simulink model "black_box_ex7"  (Simulink 7.4)
settings: Solver=VariableStepDiscrete  SolverMode=SingleTasking  StartTime=0.0  StopTime=im_size*im_size+40  RelTol=1e-3
PreLoadFcn:
  | black_box_ex7_PreLoadFcn
StopFcn:
  | black_box_ex7_StopFcn
libraries: xbsIndex_r4 x17, xbsCopyrightNotice_r4 x1
settings Model: Creator=vanessay  LastModifiedBy=douangp
settings OptimizationCC: InlineParams=on  InitFltsAndDblsToZero=on

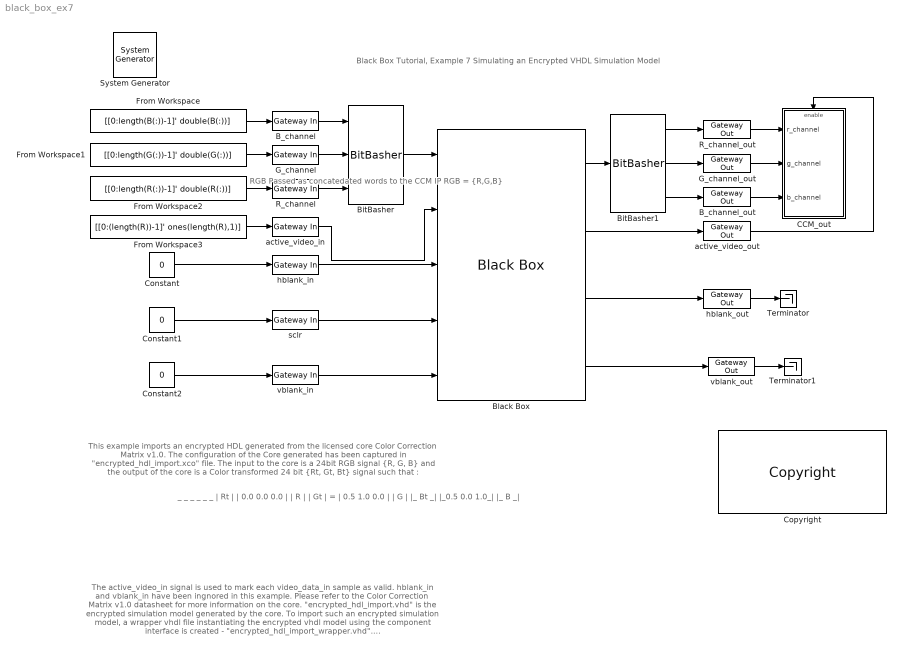
== system black_box_ex7 ==
  note: RGB Passed
      | as concatedated
      | words to the
      | CCM IP
      | RGB = {R,G,B}
  note: Black Box Tutorial, Example 7
      | Simulating an Encrypted VHDL Simulation Model
  note: This example imports an encrypted HDL generated from the licensed core Color Correction Matrix v1.0.
      | The configuration of the Core generated has been captured in "encrypted_hdl_import.xco" file. The input
      | to the core is a 24bit RGB signal {R, G, B} and the output of the core is a Color transformed 24 bit
      | {Rt, Gt, Bt} signal such that :
  note: _    _     _           _   _   _
      | |  Rt  |   | 0.0 0.0 0.0 | |  R  |
      | |  Gt  | = | 0.5 1.0 0.0 | |  G  |
      | |_ Bt _|   |_0.5 0.0 1.0_| |_ B _|
  note: The active_video_in signal is used to mark each video_data_in sample as valid. hblank_in and vblank_in
      | have been ingnored in this example. Please refer to the Color Correction Matrix v1.0 datasheet for more
      | information on the core.
      |
      | "encrypted_hdl_import.vhd" is the encrypted simulation model generated by the core. To import such an
      | encrypted simulation model, a wrapper vhdl file instantiating the encrypted vhdl model using the component
      | interface is created - "encrypted_hdl_import_wrapper.vhd". "encrypted_hdl_import_wrapper.vhd" is imported
      | using the standard Black Box import Wizard. The resulting "encrypted_hdl_import_wrapper_config.m" is
      | modified by adding the following line(line No. 103) :
      |                 this_block.addFile('encrypted_hdl_import.vhd','encrypted_hdl_import.vhd');
      | The above line instructs the SysGen netlister to netlist the encrypted file as a Separate file and not include it
      | in the consolidated HDL netlist file to allow participation of the encrypted HDL file during netlisting and simulation.
  " System Generator" : xbsIndex_r4/ System Generator  Tag=genX  SystemSampleTime=-1  xilinxfamily=spartan3adsp  part=xc3sd3400a  speed=-4  package=fg676  synthesis_tool=XST  clock_wrapper=Clock Enables  directory=./hdl  testbench=off  simulink_period=1  sysclk_period=6.6  dcm_input_clock_period=100  incr_netlist=off  trim_vbits=Everywhere in SubSystem  dbl_ovrd=According to Block Masks  core_generation=According to Block Masks  run_coregen=off  deprecated_control=off  eval_field=0  block_type=sysgen
      settings: block_version=8.2
  B_channel : xbsIndex_r4/Gateway In  arith_type=Unsigned  n_bits=8  bin_pt=0  quantization=Truncate  overflow=Wrap  period=1  dbl_ovrd=off  timing_constraint=None  locs_specified=off  LOCs={}  hdl_port=on  block_type=gatewayin
      settings: infoedit="Gateway in block.  Converts inputs of type Simulink integer, double and fixed point to  Xilinx fixed point type.<br><br>Hardware notes:  In hardware these blocks become top level input ports."  xl_area=[0, 0, 0, 0, 0, 0, 0]  block_version=VER_STRING_GOES_HERE
  B_channel_out : xbsIndex_r4/Gateway Out  hdl_port=on  timing_constraint=None  locs_specified=off  LOCs={}  block_type=gatewayout
      settings: infoedit="Gateway out block.  Converts Xilinx fixed point inputs into ouputs of type Simulink integer, double, or fixed point.<P><P>Hardware notes:  In hardware these blocks become top level output ports or are discarded, depending on how they are configured."  xl_area=[0, 0, 0, 0, 0, 0, 0]  block_version=VER_STRING_GOES_HERE
  BitBasher : xbsIndex_r4/BitBasher  bitexpr=|  display_expr=off  sr_1=1  arith_type1=Unsigned  bin_pt1=0  sr_2=2  arith_type2=Unsigned  bin_pt2=0  sr_3=3  arith_type3=Unsigned  bin_pt3=0  sr_4=4  arith_type4=Unsigned  bin_pt4=0  dbl_ovrd=off  block_type=bitbasher
      | <!DOCTYPE HTML PUBLIC "-//W3C//DTD HTML 4.0//EN" "http://www.w3.org/TR/REC-html40/strict.dtd">
      | <html><head><meta name="qrichtext" content="1" /><style type="text/css">
      | p, li { white-space: pre-wrap; }
      | </style></head><body style=" font-family:'MS Shell Dlg 2'; font-size:8.25pt; font-weight:400; font-style:normal;">
      | <p style=" margin-top:12px; margin-bottom:12px; margin-left:0px; margin-right:0px; -qt-block-indent:0; text-indent:0px; font-family:'MS Shell Dlg'; font-size:8pt;">RGB={R,G,B}</p></body></html>
      settings: block_version=11.3
  BitBasher1 : xbsIndex_r4/BitBasher  bitexpr=|  display_expr=off  sr_1=1  arith_type1=Unsigned  bin_pt1=0  sr_2=2  arith_type2=Unsigned  bin_pt2=0  sr_3=3  arith_type3=Unsigned  bin_pt3=0  sr_4=4  arith_type4=Unsigned  bin_pt4=0  dbl_ovrd=off  block_type=bitbasher
      | <!DOCTYPE HTML PUBLIC "-//W3C//DTD HTML 4.0//EN" "http://www.w3.org/TR/REC-html40/strict.dtd">
      | <html><head><meta name="qrichtext" content="1" /><style type="text/css">
      | p, li { white-space: pre-wrap; }
      | </style></head><body style=" font-family:'MS Shell Dlg 2'; font-size:8.25pt; font-weight:400; font-style:normal;">
      | <p style=" margin-top:12px; margin-bottom:12px; margin-left:0px; margin-right:0px; -qt-block-indent:0; text-indent:0px; font-family:'MS Shell Dlg'; font-size:8pt;">R={RGB[23:16]}<br />G={RGB[15:8]}<br />B={RGB[7:0]}</p></body></html>
      settings: block_version=11.3
  Black Box : xbsIndex_r4/Black Box  init_code=encrypted_hdl_import_wrapper_config  sim_method=ISE Simulator  verbose=off  block_type=blackbox2
      settings: block_version=11.3
  CCM_out : Subsystem  TreatAsAtomicUnit=on
  Constant : Constant  Value=0  OutDataType=sfix(16)  OutScaling=2^0
  Constant1 : Constant  Value=0  OutDataType=sfix(16)  OutScaling=2^0
  Constant2 : Constant  Value=0  OutDataType=sfix(16)  OutScaling=2^0
  Copyright : xbsCopyrightNotice_r4/Copyright  copyrighttext="Copyright (c) 2010  by  Xilinx, Inc. All rights reserved.<br><br>This file contains proprietary, confidential information of Xilinx, Inc., is distributed under licensefrom Xilinx, Inc., and may be used, copied and/or disclosed only pursuant to the terms of a valid licenseagreement with Xilinx, Inc. Xilinx hereby grants you a license to use this file solely for design,simulation, implementation and creation of design files limited to Xilinx devices or technologies. Use with non-Xilinx devices or technologies is expressly prohibited and immediately terminates your license unless covered by a separate agreement.<br><br>Xilinx is providing this design, code, or information \"as-is\" solely for use in developing programs and solutions for Xilinx devices, with no obligation on the part of Xilinx to provide support. By providingthis design, code, or information as one possible implementation of this feature, application or standard,Xilinx is making no representation that this implementation is free from any claims of infringement. Youare responsible for obtaining any rights you may require for your implementation. Xilinx expressly disclaimsany warranty whatsoever with respect to the adequacy of the implementation, including but not limited to anywarranties or representations that this implementation is free from claims of infringement, implied warrantiesof merchantability or fitness for a particular purpose.<br><br>Xilinx products are not intended for use in life support appliances, devices, or systems. Use in such applications is expressly prohibited.<br><br>Any modifications that are made to the Source Code are done at the user's sole risk and will be unsupported.<br><br>This copyright and support notice must be retained as part of this text at all times. (c) Copyright 1995-2010 Xilinx, Inc. All rights reserved."  block_type=copyright
      settings: block_version=10.1.3
      settings: infoedit=|
      | Copyright(C) 2008 by  Xilinx, Inc. All rights reserved.<br>
      | <br>
      | This file contains proprietary, confidential information of Xilinx, Inc., is distributed under license
      | from Xilinx, Inc., and may be used, copied and/or disclosed only pursuant to the terms of a valid license
      | agreement with Xilinx, Inc. Xilinx hereby grants you a license to use this file solely for design,
      | simulation, implementation and creation of design files limited to Xilinx devices or technologies. Use
      | with non-Xilinx devices or technologies is expressly prohibited and immediately terminates your license
      | unless covered by a separate agreement.<br>
      | <br>
      | Xilinx is providing this design, code, or information "as-is" solely for use in developing programs and
      | solutions for Xilinx devices, with no obligation on the part of Xilinx to provide support. By providing
      | this design, code, or information as one possible implementation of this feature, application or standard,
      | Xilinx is making no representation that this implementation is free from any claims of infringement. You
      | are responsible for obtaining any rights you may require for your implementation. Xilinx expressly disclaims
      | any warranty whatsoever with respect to the adequacy of the implementation, including but not limited to any
      | warranties or representations that this implementation is free from claims of infringement, implied warranties
      | of merchantability or fitness for a particular purpose.<br>
      | <br>
      | Xilinx products are not intended for use in life support appliances, devices, or systems. Use in such
      | applications is expressly prohibited.<br>
      | <br>
      | Any modifications that are made to the Source Code are done at the user's sole risk and will be unsupported.<br>
      | <br>
      | This copyright and support notice must be retained as part of this text at all times.
      | (c) Copyright 1995-2008 Xilinx, Inc. All rights reserved.
  From Workspace : FromWorkspace  VariableName=[[0:length(B(:))-1]' double(B(:))]  SampleTime=1
  From Workspace1 : FromWorkspace  VariableName=[[0:length(G(:))-1]' double(G(:))]  SampleTime=1
  From Workspace2 : FromWorkspace  VariableName=[[0:length(R(:))-1]' double(R(:))]  SampleTime=1
  From Workspace3 : FromWorkspace  VariableName=[[0:(length(R))-1]' ones(length(R),1)]  SampleTime=1  OutputAfterFinalValue=Setting to zero
  G_channel : xbsIndex_r4/Gateway In  arith_type=Unsigned  n_bits=8  bin_pt=0  quantization=Truncate  overflow=Wrap  period=1  dbl_ovrd=off  timing_constraint=None  locs_specified=off  LOCs={}  hdl_port=on  block_type=gatewayin
      settings: infoedit="Gateway in block.  Converts inputs of type Simulink integer, double and fixed point to  Xilinx fixed point type.<br><br>Hardware notes:  In hardware these blocks become top level input ports."  xl_area=[0, 0, 0, 0, 0, 0, 0]  block_version=VER_STRING_GOES_HERE
  G_channel_out : xbsIndex_r4/Gateway Out  hdl_port=on  timing_constraint=None  locs_specified=off  LOCs={}  block_type=gatewayout
      settings: infoedit="Gateway out block.  Converts Xilinx fixed point inputs into ouputs of type Simulink integer, double, or fixed point.<P><P>Hardware notes:  In hardware these blocks become top level output ports or are discarded, depending on how they are configured."  xl_area=[0, 0, 0, 0, 0, 0, 0]  block_version=VER_STRING_GOES_HERE
  R_channel : xbsIndex_r4/Gateway In  arith_type=Unsigned  n_bits=8  bin_pt=0  quantization=Truncate  overflow=Wrap  period=1  dbl_ovrd=off  timing_constraint=None  locs_specified=off  LOCs={}  hdl_port=on  block_type=gatewayin
      settings: infoedit="Gateway in block.  Converts inputs of type Simulink integer, double and fixed point to  Xilinx fixed point type.<br><br>Hardware notes:  In hardware these blocks become top level input ports."  xl_area=[0, 0, 0, 0, 0, 0, 0]  block_version=VER_STRING_GOES_HERE
  R_channel_out : xbsIndex_r4/Gateway Out  hdl_port=on  timing_constraint=None  locs_specified=off  LOCs={}  block_type=gatewayout
      settings: infoedit="Gateway out block.  Converts Xilinx fixed point inputs into ouputs of type Simulink integer, double, or fixed point.<P><P>Hardware notes:  In hardware these blocks become top level output ports or are discarded, depending on how they are configured."  xl_area=[0, 0, 0, 0, 0, 0, 0]  block_version=VER_STRING_GOES_HERE
  Terminator : Terminator
  Terminator1 : Terminator
  active_video_in : xbsIndex_r4/Gateway In  arith_type=Unsigned  n_bits=1  bin_pt=0  quantization=Truncate  overflow=Wrap  period=1  dbl_ovrd=off  timing_constraint=None  locs_specified=off  LOCs={}  hdl_port=on  block_type=gatewayin
      settings: infoedit="Gateway in block.  Converts inputs of type Simulink integer, double and fixed point to  Xilinx fixed point type.<br><br>Hardware notes:  In hardware these blocks become top level input ports."  xl_area=[0, 0, 0, 0, 0, 0, 0]  block_version=VER_STRING_GOES_HERE
  active_video_out : xbsIndex_r4/Gateway Out  hdl_port=on  timing_constraint=None  locs_specified=off  LOCs={}  block_type=gatewayout
      settings: infoedit="Gateway out block.  Converts Xilinx fixed point inputs into ouputs of type Simulink integer, double, or fixed point.<P><P>Hardware notes:  In hardware these blocks become top level output ports or are discarded, depending on how they are configured."  xl_area=[0, 0, 0, 0, 0, 0, 0]  block_version=VER_STRING_GOES_HERE
  hblank_in : xbsIndex_r4/Gateway In  arith_type=Unsigned  n_bits=1  bin_pt=0  quantization=Truncate  overflow=Wrap  period=1  dbl_ovrd=off  timing_constraint=None  locs_specified=off  LOCs={}  hdl_port=on  block_type=gatewayin
      settings: infoedit="Gateway in block.  Converts inputs of type Simulink integer, double and fixed point to  Xilinx fixed point type.<br><br>Hardware notes:  In hardware these blocks become top level input ports."  xl_area=[0, 0, 0, 0, 0, 0, 0]  block_version=VER_STRING_GOES_HERE
  hblank_out : xbsIndex_r4/Gateway Out  hdl_port=on  timing_constraint=None  locs_specified=off  LOCs={}  block_type=gatewayout
      settings: infoedit="Gateway out block.  Converts Xilinx fixed point inputs into ouputs of type Simulink integer, double, or fixed point.<P><P>Hardware notes:  In hardware these blocks become top level output ports or are discarded, depending on how they are configured."  xl_area=[0, 0, 0, 0, 0, 0, 0]  block_version=VER_STRING_GOES_HERE
  sclr : xbsIndex_r4/Gateway In  arith_type=Unsigned  n_bits=1  bin_pt=0  quantization=Truncate  overflow=Wrap  period=1  dbl_ovrd=off  timing_constraint=None  locs_specified=off  LOCs={}  hdl_port=on  block_type=gatewayin
      settings: infoedit="Gateway in block.  Converts inputs of type Simulink integer, double and fixed point to  Xilinx fixed point type.<br><br>Hardware notes:  In hardware these blocks become top level input ports."  xl_area=[0, 0, 0, 0, 0, 0, 0]  block_version=VER_STRING_GOES_HERE
  vblank_in : xbsIndex_r4/Gateway In  arith_type=Unsigned  n_bits=1  bin_pt=0  quantization=Truncate  overflow=Wrap  period=1  dbl_ovrd=off  timing_constraint=None  locs_specified=off  LOCs={}  hdl_port=on  block_type=gatewayin
      settings: infoedit="Gateway in block.  Converts inputs of type Simulink integer, double and fixed point to  Xilinx fixed point type.<br><br>Hardware notes:  In hardware these blocks become top level input ports."  xl_area=[0, 0, 0, 0, 0, 0, 0]  block_version=VER_STRING_GOES_HERE
  vblank_out : xbsIndex_r4/Gateway Out  hdl_port=on  timing_constraint=None  locs_specified=off  LOCs={}  block_type=gatewayout
      settings: infoedit="Gateway out block.  Converts Xilinx fixed point inputs into ouputs of type Simulink integer, double, or fixed point.<P><P>Hardware notes:  In hardware these blocks become top level output ports or are discarded, depending on how they are configured."  xl_area=[0, 0, 0, 0, 0, 0, 0]  block_version=VER_STRING_GOES_HERE
  wires:
  Black Box/4 -> vblank_out/1
  Black Box/3 -> hblank_out/1
  Black Box/2 -> active_video_out/1
  B_channel/1 -> BitBasher/1
  G_channel/1 -> BitBasher/2
  R_channel/1 -> BitBasher/3
  From Workspace/1 -> B_channel/1
  From Workspace1/1 -> G_channel/1
  From Workspace2/1 -> R_channel/1
  Black Box/1 -> BitBasher1/1
  BitBasher1/1 -> R_channel_out/1
  BitBasher1/2 -> G_channel_out/1
  BitBasher1/3 -> B_channel_out/1
  Constant/1 -> hblank_in/1
  Constant1/1 -> sclr/1
  Constant2/1 -> vblank_in/1
  BitBasher/1 -> Black Box/1
  vblank_in/1 -> Black Box/5
  sclr/1 -> Black Box/4
  hblank_in/1 -> Black Box/3
  From Workspace3/1 -> active_video_in/1
  active_video_in/1 -> Black Box/2
  R_channel_out/1 -> CCM_out/1(r_channel)
  G_channel_out/1 -> CCM_out/2(g_channel)
  B_channel_out/1 -> CCM_out/3(b_channel)
  hblank_out/1 -> Terminator/1
  vblank_out/1 -> Terminator1/1
  active_video_out/1 -> CCM_out/Enable

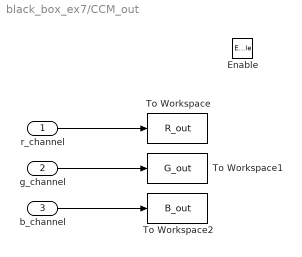
== system black_box_ex7/CCM_out ==
  r_channel : Inport  OutDataType=sfix(16)  OutScaling=2^0
  g_channel : Inport  Port=2  OutDataType=sfix(16)  OutScaling=2^0
  b_channel : Inport  Port=3  OutDataType=sfix(16)  OutScaling=2^0
  Enable : EnablePort
  To Workspace : ToWorkspace  VariableName=R_out  SampleTime=-1  SaveFormat=Array
  To Workspace1 : ToWorkspace  VariableName=G_out  SampleTime=-1  SaveFormat=Array
  To Workspace2 : ToWorkspace  VariableName=B_out  SampleTime=-1  SaveFormat=Array
  wires:
  r_channel/1 -> To Workspace/1
  g_channel/1 -> To Workspace1/1
  b_channel/1 -> To Workspace2/1
